simulink model "lr3model"  (R2020a)
settings: Solver=FixedStepAuto  StartTime=0.0  StopTime=50  FixedStep=1e-4  RelTol=1e-3
undefined symbols (not defined in the file or in its folder): magnitude
settings Model: Creator=Vasiliy  LastModifiedBy=Ксения
settings DebuggingCC: AlgebraicLoopMsg=none  SFMachineParentedDataDiag=error

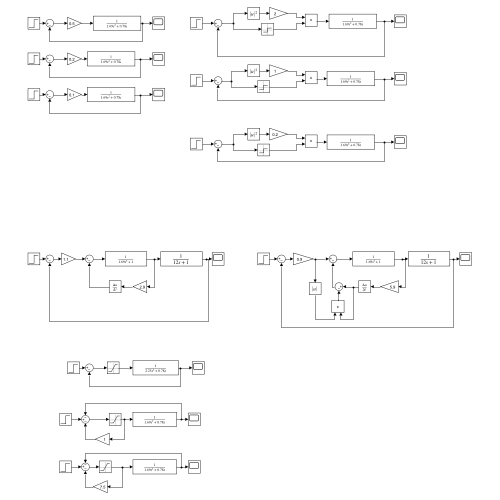
[thumbnail: Simulink's stored preview of the top-level diagram]
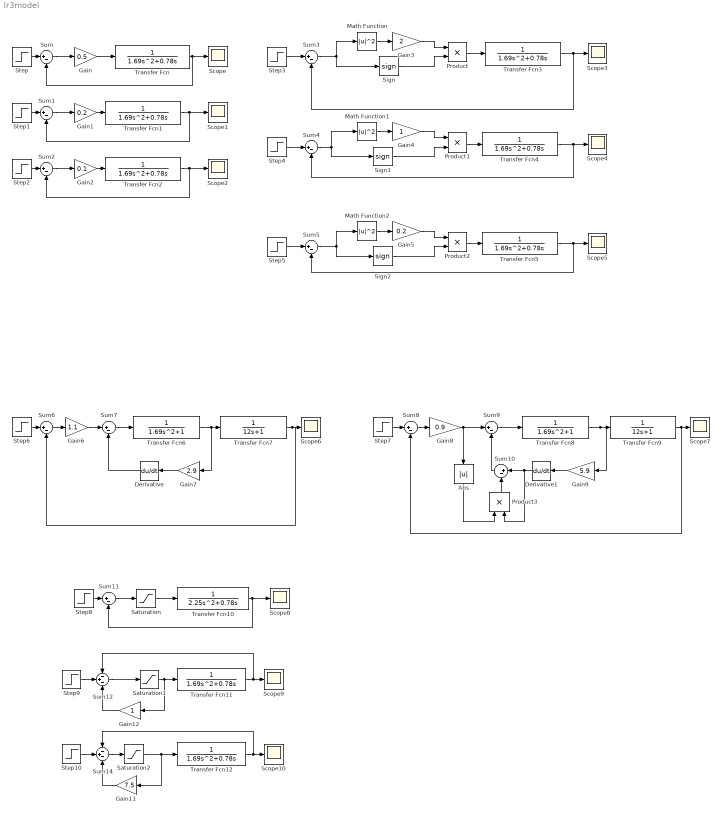
== system lr3model ==
  Abs : Abs
  Derivative : Derivative
  Derivative1 : Derivative
  Gain : Gain  Gain=0.5
  Gain1 : Gain  Gain=0.2
  Gain11 : Gain  Gain=7.5
  Gain12 : Gain
  Gain2 : Gain  Gain=0.1
  Gain3 : Gain  Gain=2
  Gain4 : Gain
  Gain5 : Gain  Gain=0.2
  Gain6 : Gain  Gain=1.1
  Gain7 : Gain  Gain=2.9
  Gain8 : Gain  Gain=0.9
  Gain9 : Gain  Gain=5.9
  Math Function : Math  Operator=magnitude^2  SaturateOnIntegerOverflow=on
  Math Function1 : Math  Operator=magnitude^2  SaturateOnIntegerOverflow=on
  Math Function2 : Math  Operator=magnitude^2  SaturateOnIntegerOverflow=on
  Product{,1..3} (4 alike) : Product
  Saturation : Saturate
  Saturation1 : Saturate
  Saturation2 : Saturate
  Scope{,1..10} (11 alike) : Scope
  Sign : Signum
  Sign1 : Signum
  Sign2 : Signum
  Step{,1..10} (11 alike) : Step  SampleTime=0
  Sum{,1..11} (12 alike) : Sum  Inputs=|+-
  Sum12 : Sum  Inputs=-+-
  Sum14 : Sum  Inputs=-+-
  Transfer Fcn{,1..5,11..12} (8 alike) : TransferFcn  Denominator=[1.69 0.78 0]
  Transfer Fcn10 : TransferFcn  Denominator=[2.25 0.78 0]
  Transfer Fcn6 : TransferFcn  Denominator=[1.69 0 1]
  Transfer Fcn7 : TransferFcn  Denominator=[12 1]
  Transfer Fcn8 : TransferFcn  Denominator=[1.69 0 1]
  Transfer Fcn9 : TransferFcn  Denominator=[12 1]
  wires:
  Transfer Fcn/1 -> Sum/2, Scope/1
  Step/1 -> Sum/1
  Sum/1 -> Gain/1
  Gain/1 -> Transfer Fcn/1
  Step1/1 -> Sum1/1
  Gain1/1 -> Transfer Fcn1/1
  Sum1/1 -> Gain1/1
  Transfer Fcn1/1 -> Scope1/1, Sum1/2
  Step2/1 -> Sum2/1
  Sum2/1 -> Gain2/1
  Transfer Fcn2/1 -> Scope2/1, Sum2/2
  Sum3/1 -> Math Function/1, Sign/1
  Sign/1 -> Product/2
  Step3/1 -> Sum3/1
  Transfer Fcn3/1 -> Sum3/2, Scope3/1
  Gain4/1 -> Product1/1
  Sum4/1 -> Math Function1/1, Sign1/1
  Sign1/1 -> Product1/2
  Step4/1 -> Sum4/1
  Transfer Fcn4/1 -> Sum4/2, Scope4/1
  Gain5/1 -> Product2/1
  Sum5/1 -> Math Function2/1, Sign2/1
  Sign2/1 -> Product2/2
  Step5/1 -> Sum5/1
  Transfer Fcn5/1 -> Sum5/2, Scope5/1
  Sum6/1 -> Gain6/1
  Step6/1 -> Sum6/1
  Transfer Fcn6/1 -> Transfer Fcn7/1, Gain7/1
  Gain6/1 -> Sum7/1
  Sum7/1 -> Transfer Fcn6/1
  Derivative/1 -> Sum7/2
  Gain7/1 -> Derivative/1
  Transfer Fcn7/1 -> Scope6/1, Sum6/2
  Gain8/1 -> Abs/1, Sum9/1
  Gain9/1 -> Derivative1/1
  Derivative1/1 -> Sum10/1, Product3/2
  Sum9/1 -> Transfer Fcn8/1
  Transfer Fcn9/1 -> Scope7/1, Sum8/2
  Sum8/1 -> Gain8/1
  Transfer Fcn8/1 -> Transfer Fcn9/1, Gain9/1
  Step7/1 -> Sum8/1
  Abs/1 -> Product3/1
  Product3/1 -> Sum10/2
  Sum10/1 -> Sum9/2
  Step8/1 -> Sum11/1
  Saturation/1 -> Transfer Fcn10/1
  Sum11/1 -> Saturation/1
  Transfer Fcn10/1 -> Scope8/1, Sum11/2
  Transfer Fcn11/1 -> Sum12/1, Scope9/1
  Saturation2/1 -> Transfer Fcn12/1, Gain11/1
  Transfer Fcn12/1 -> Scope10/1, Sum14/1
  Sum14/1 -> Saturation2/1
  Gain11/1 -> Sum14/3
  Step9/1 -> Sum12/2
  Sum12/1 -> Saturation1/1
  Step10/1 -> Sum14/2
  Math Function/1 -> Gain3/1
  Gain3/1 -> Product/1
  Math Function1/1 -> Gain4/1
  Math Function2/1 -> Gain5/1
  Gain12/1 -> Sum12/3
  Saturation1/1 -> Gain12/1, Transfer Fcn11/1
  Gain2/1 -> Transfer Fcn2/1
  Product/1 -> Transfer Fcn3/1
  Product1/1 -> Transfer Fcn4/1
  Product2/1 -> Transfer Fcn5/1
